simulink model "udp_receiver"  (R2018b)
settings: Solver=VariableStepAuto  StartTime=0.0  StopTime=inf  RelTol=1e-3
libraries: dspnetwork x1
settings Model: Creator=nicolai  LastModifiedBy=nicolai

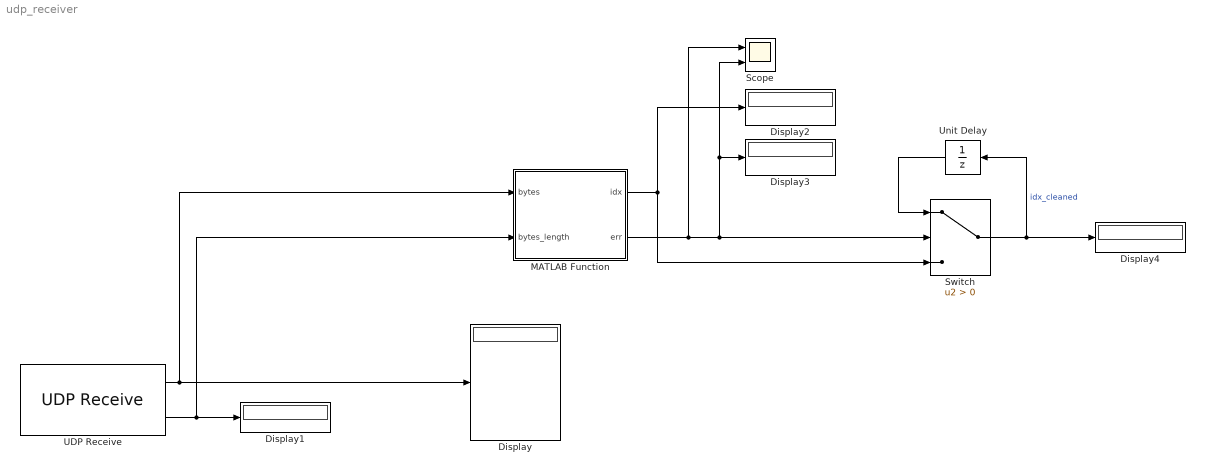
== system udp_receiver ==
  Display{,1..4} (5 alike) : Display
  MATLAB Function : MATLAB Function  TreatAsAtomicUnit=on
  Scope : Scope  NumInputPorts=2
  Switch : Switch  Criteria=u2 > Threshold
  UDP Receive : dspnetwork/UDP Receive  localURL='0.0.0.0'  localPort=25000  remoteURL='0.0.0.0'  remotePort=-1  recvBufferSize=8192  dims=5  signalDatatype=uint8  isVarSize=off  showBlockingTime=off  blockingTime=0  sampletime=1  blockPlatform=[]
      settings: SourceProductName=DSP System Toolbox  SourceProductBaseCode=DS
  Unit Delay : UnitDelay  SampleTime=-1
  wires:
  UDP Receive/1 -> MATLAB Function/1(bytes), Display/1
  UDP Receive/2 -> MATLAB Function/2(bytes_length), Display1/1
  MATLAB Function/1(idx) -> Display2/1, Switch/3
  MATLAB Function/2(err) -> Scope/1, Switch/2, Scope/2, Display3/1
  Switch/1 -> Unit Delay/1, Display4/1  "idx_cleaned"
  Unit Delay/1 -> Switch/1

== matlab function udp_receiver/MATLAB Function ==
  data: bytes input; idx output; bytes_length input; err output
function [idx,err] = fcn(bytes, bytes_length)

[idx,err]=microbuf.check_array(bytes, length(bytes), 3, 1);
